simulink model "sim_simx"  (R2020b)
settings: Solver=VariableStepAuto  StartTime=0.0  StopTime=10.0  RelTol=1e-3
PreLoadFcn:
  | k;
values from neighbouring files (symbols this model uses):
  CF = 1300    [importlocation.m]    (also in k.m)
  iBig = 30    [importlocation.m]    (also in k.m)
  Km = 42.9e-3    (= 0.0429)    [importlocation.m]    (also in k.m)
  Lw = 0.514e-3    (= 0.000514)    [importlocation.m]    (also in k.m)
  Rw = 2.68    [importlocation.m]    (also in k.m)
libraries: cstblocks x2, pid_lib x2, simulink x2
settings Model: PreStartFcn=k;  Creator=28217  LastModifiedBy=28217

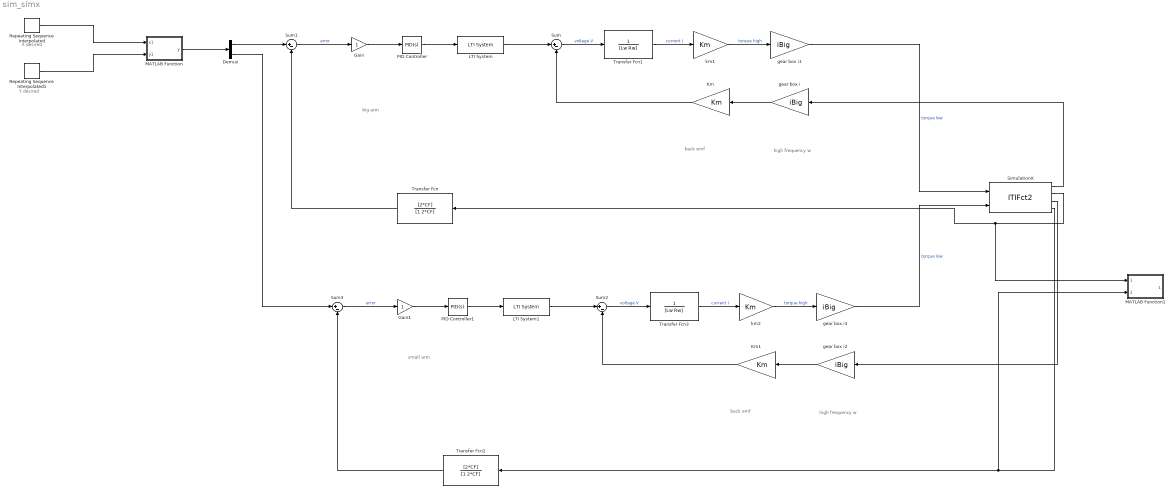
== system sim_simx ==
  note: Y desired
  note: X desired
  note: small arm
  note: big arm
  note: back emf
  note: high frequency w
  note: back emf
  note: high frequency w
  Demux : Demux  Outputs=2
  Gain : Gain
  Gain1 : Gain
  Km : Gain  Gain=Km
  Km1 : Gain  Gain=Km
  LTI System : cstblocks/LTI System  sys=ampTF  IC=[]
  LTI System1 : cstblocks/LTI System  sys=ampTF  IC=[]
  MATLAB Function : MATLAB Function  TreatAsAtomicUnit=on
  MATLAB Function1 : MATLAB Function  TreatAsAtomicUnit=on
  PID Controller : pid_lib/PID Controller  Controller=PID  Form=Parallel  TimeDomain=Continuous-time  UseExternalTs=off  SampleTime=-1  IntegratorMethod=Forward Euler  FilterMethod=Forward Euler  ControllerParametersSource=internal  P=1  I=0  D=0  UseFilter=on  N=100  TunerSelectOption=Transfer Function Based (PID Tuner App)  InitialConditionSource=internal  InitialConditionForIntegrator=0  InitialConditionForFilter=0  DifferentiatorICPrevScaledInput=0  ExternalReset=none  TrackingMode=off  Kt=1  LimitOutput=off  SatLimitsSource=internal  UpperSaturationLimit=inf  LowerSaturationLimit=-inf  LinearizeAsGain=on  AntiWindupMode=none  Kb=1  POutMin=[]  POutMax=[]  IOutMin=[]  IOutMax=[]  DOutMin=[]  DOutMax=[]  NOutMin=[]  NOutMax=[]  SumOutMin=[]  SumOutMax=[]  SaturationOutMin=[]  SaturationOutMax=[]  PParamMin=[]  PParamMax=[]  IParamMin=[]  IParamMax=[]  DParamMin=[]  DParamMax=[]  NParamMin=[]  NParamMax=[]  KbParamMin=[]  KbParamMax=[]  KtParamMin=[]  KtParamMax=[]  KbOutMin=[]  KbOutMax=[]  KtOutMin=[]  KtOutMax=[]  IntegratorOutMin=[]  IntegratorOutMax=[]  FilterOutMin=[]  FilterOutMax=[]  SumI1OutMin=[]  SumI1OutMax=[]  SumI2OutMin=[]  SumI2OutMax=[]  SumI3OutMin=[]  SumI3OutMax=[]  SumI4OutMin=[]  SumI4OutMax=[]  SumDOutMin=[]  SumDOutMax=[]  DifferentiatorOutMin=[]  DifferentiatorOutMax=[]  FilterDiffOutCoefMin=[]  FilterDiffOutCoefMax=[]  ReciprocalOutMin=[]  ReciprocalOutMax=[]  SumDenOutMin=[]  SumDenOutMax=[]  SumNumOutMin=[]  SumNumOutMax=[]  DivideOutMin=[]  DivideOutMax=[]  UdiffTsProdOutMin=[]  UdiffTsProdOutMax=[]  NTsProdOutMin=[]  NTsProdOutMax=[]  UintegralTsProdOutMin=[]  UintegralTsProdOutMax=[]  UngainTsProdOutMin=[]  UngainTsProdOutMax=[]  IntegratorContinuousStateAttributes=''  IntegratorStateMustResolveToSignalObject=off  IntegratorRTWStateStorageClass=Auto  FilterContinuousStateAttributes=''  FilterStateMustResolveToSignalObject=off  FilterRTWStateStorageClass=Auto  ParallelPVariant=InternalParameters  IdealPVariant=Disabled  IVariant=InternalParameters  DVariant=InternalParameters  IntegratorVariant=Continuous  SatVariant=Disabled  AWVariant=Passthrough  PCopyVariant=Disabled  TRVariant=Disabled  FdbkBlocksVariant=Forward  IdealPFdbkVariant=Disabled  SatFdbkVariant=Disabled  DerivativeFilterVariant=ContFilter  NVariant=InternalParameters  NCopyVariant=Disabled  FilterICVariant=InternalICsFilter  IntegratorICVariant=InternalICs  ExternalResetVariant=Disabled  TRSumVariant=Passthrough  SumFdbkVariant=Disabled  SumVariant=Sum_PID  TsampFilterVariant=InternalTs  TsampNgainVariant=Passthrough  TsampIntegralVariant=Passthrough  ExternalSaturationOutDataTypeStr=Inherit: Same as second input
  PID Controller1 : pid_lib/PID Controller  Controller=PID  Form=Parallel  TimeDomain=Continuous-time  UseExternalTs=off  SampleTime=-1  IntegratorMethod=Forward Euler  FilterMethod=Forward Euler  ControllerParametersSource=internal  P=1  I=0  D=0  UseFilter=on  N=100  TunerSelectOption=Transfer Function Based (PID Tuner App)  InitialConditionSource=internal  InitialConditionForIntegrator=0  InitialConditionForFilter=0  DifferentiatorICPrevScaledInput=0  ExternalReset=none  TrackingMode=off  Kt=1  LimitOutput=off  SatLimitsSource=internal  UpperSaturationLimit=inf  LowerSaturationLimit=-inf  LinearizeAsGain=on  AntiWindupMode=none  Kb=1  POutMin=[]  POutMax=[]  IOutMin=[]  IOutMax=[]  DOutMin=[]  DOutMax=[]  NOutMin=[]  NOutMax=[]  SumOutMin=[]  SumOutMax=[]  SaturationOutMin=[]  SaturationOutMax=[]  PParamMin=[]  PParamMax=[]  IParamMin=[]  IParamMax=[]  DParamMin=[]  DParamMax=[]  NParamMin=[]  NParamMax=[]  KbParamMin=[]  KbParamMax=[]  KtParamMin=[]  KtParamMax=[]  KbOutMin=[]  KbOutMax=[]  KtOutMin=[]  KtOutMax=[]  IntegratorOutMin=[]  IntegratorOutMax=[]  FilterOutMin=[]  FilterOutMax=[]  SumI1OutMin=[]  SumI1OutMax=[]  SumI2OutMin=[]  SumI2OutMax=[]  SumI3OutMin=[]  SumI3OutMax=[]  SumI4OutMin=[]  SumI4OutMax=[]  SumDOutMin=[]  SumDOutMax=[]  DifferentiatorOutMin=[]  DifferentiatorOutMax=[]  FilterDiffOutCoefMin=[]  FilterDiffOutCoefMax=[]  ReciprocalOutMin=[]  ReciprocalOutMax=[]  SumDenOutMin=[]  SumDenOutMax=[]  SumNumOutMin=[]  SumNumOutMax=[]  DivideOutMin=[]  DivideOutMax=[]  UdiffTsProdOutMin=[]  UdiffTsProdOutMax=[]  NTsProdOutMin=[]  NTsProdOutMax=[]  UintegralTsProdOutMin=[]  UintegralTsProdOutMax=[]  UngainTsProdOutMin=[]  UngainTsProdOutMax=[]  IntegratorContinuousStateAttributes=''  IntegratorStateMustResolveToSignalObject=off  IntegratorRTWStateStorageClass=Auto  FilterContinuousStateAttributes=''  FilterStateMustResolveToSignalObject=off  FilterRTWStateStorageClass=Auto  ParallelPVariant=InternalParameters  IdealPVariant=Disabled  IVariant=InternalParameters  DVariant=InternalParameters  IntegratorVariant=Continuous  SatVariant=Disabled  AWVariant=Passthrough  PCopyVariant=Disabled  TRVariant=Disabled  FdbkBlocksVariant=Forward  IdealPFdbkVariant=Disabled  SatFdbkVariant=Disabled  DerivativeFilterVariant=ContFilter  NVariant=InternalParameters  NCopyVariant=Disabled  FilterICVariant=InternalICsFilter  IntegratorICVariant=InternalICs  ExternalResetVariant=Disabled  TRSumVariant=Passthrough  SumFdbkVariant=Disabled  SumVariant=Sum_PID  TsampFilterVariant=InternalTs  TsampNgainVariant=Passthrough  TsampIntegralVariant=Passthrough  ExternalSaturationOutDataTypeStr=Inherit: Same as second input
  Repeating Sequence Interpolated : simulink/Sources/Repeating Sequence Interpolated  OutValues=[3 1 4 2 1].'  TimeValues=[0 0.1 0.5 0.6 1].'  LookUpMeth=Interpolation-Use End Values  tsamp=0.01  OutMin=[]  OutMax=[]  OutDataTypeStr=double  OutputDataTypeScalingMode=double  OutDataType=fixdt(0,8)  OutScaling=2^-10
  Repeating Sequence Interpolated1 : simulink/Sources/Repeating Sequence Interpolated  OutValues=[3 1 4 2 1].'  TimeValues=[0 0.1 0.5 0.6 1].'  LookUpMeth=Interpolation-Use End Values  tsamp=0.01  OutMin=[]  OutMax=[]  OutDataTypeStr=double  OutputDataTypeScalingMode=double  OutDataType=fixdt(0,8)  OutScaling=2^-10
  "SimulationX " : S-Function  FunctionName=ITIFct2  Parameters=ip, port, ts, nIn, nOut  SFunctionDeploymentMode=off  EnableBusSupport=off  mask{ip='localhost', port=4097, ts=0.001, nIn=2, nOut=4}
      mask prompts: ip "Address: ip"; port "Port Number: port [-]"; ts "Communication Step Size: ts [s]"; nIn "Input Vector Dimension (to SimulationX): nIn [-]"; nOut "Output Vector Dimension (from SimulationX): nOut [-]"
      mask help: Coupling Element
  Sum{,1..3} (4 alike) : Sum  Inputs=|+-
  Transfer Fcn : TransferFcn  Numerator=[2*CF]  Denominator=[1 2*CF]
  Transfer Fcn1 : TransferFcn  Denominator=[Lw Rw]
  Transfer Fcn2 : TransferFcn  Numerator=[2*CF]  Denominator=[1 2*CF]
  Transfer Fcn3 : TransferFcn  Denominator=[Lw Rw]
  gear box i{,1..3} (4 alike) : Gain  Gain=iBig
  km1 : Gain  Gain=Km
  km2 : Gain  Gain=Km
  wires:
  Transfer Fcn1/1 -> km1/1  "current I"
  km1/1 -> gear box i1/1  "torque high"
  Sum/1 -> Transfer Fcn1/1  "voltage V"
  Km/1 -> Sum/2
  gear box i/1 -> Km/1
  PID Controller/1 -> LTI System/1
  Sum1/1 -> Gain/1  "error"
  Transfer Fcn/1 -> Sum1/2
  Gain/1 -> PID Controller/1
  LTI System/1 -> Sum/1
  LTI System1/1 -> Sum2/1
  Km1/1 -> Sum2/2
  Sum3/1 -> Gain1/1  "error"
  PID Controller1/1 -> LTI System1/1
  Gain1/1 -> PID Controller1/1
  Transfer Fcn2/1 -> Sum3/2
  Transfer Fcn3/1 -> km2/1  "current I"
  Sum2/1 -> Transfer Fcn3/1  "voltage V"
  km2/1 -> gear box i3/1  "torque high"
  gear box i2/1 -> Km1/1
  gear box i1/1 -> "SimulationX "/1  "torque low"
  gear box i3/1 -> "SimulationX "/2  "torque low"
  MATLAB Function/1(y) -> Demux/1
  Demux/1 -> Sum1/1
  Demux/2 -> Sum3/1
  "SimulationX "/1 -> gear box i/1
  "SimulationX "/2 -> MATLAB Function1/1(angle1), Transfer Fcn/1
  "SimulationX "/3 -> gear box i2/1
  "SimulationX "/4 -> MATLAB Function1/2(angle2), Transfer Fcn2/1
  Repeating Sequence Interpolated/1 -> MATLAB Function/1(x1)
  Repeating Sequence Interpolated1/1 -> MATLAB Function/2(y1)

== matlab function sim_simx/MATLAB Function ==
  data: x1 input; y output; y1 input
function y = fcn(x1,y1)
arm1 = 0.25
arm2 = 0.35

sx = x1;
sy = y1;
angle2 = -acos((sx^2 + sy^2 - arm1^2 - arm2^2 )/(2*arm1*arm2))  %sign could be positive or negative 
b2 = (sx^2 + sy^2 - arm1^2 - arm2^2)/(2 * arm1 * arm2);
s2 = sqrt(1-b2^2);
angle1 = atan2(arm2^2*s2*x1+(arm1+arm2*b2)*sy,(arm1+arm2*b2)*sx-arm2*s2*sy);


y = [angle1,angle2];

== matlab function sim_simx/MATLAB Function1 ==
  data: angle1 input; location output; angle2 input
function location = fcn(angle1,angle2)
arm1 = 0.25
arm2 = 0.35

x1 = arm1*cos(angle1) + arm2*cos(angle1+angle2);
y1 = arm1*sin(angle1) + arm2*sin(angle1+angle2);

location = [x1,y1];
end
